simulink subsystem "controller_change"  (R2022b)
settings: Solver=VariableStepAuto  StartTime=0.0  StopTime=10.0  RelTol=1e-3
settings Model: Creator=Edp  LastModifiedBy=Edp

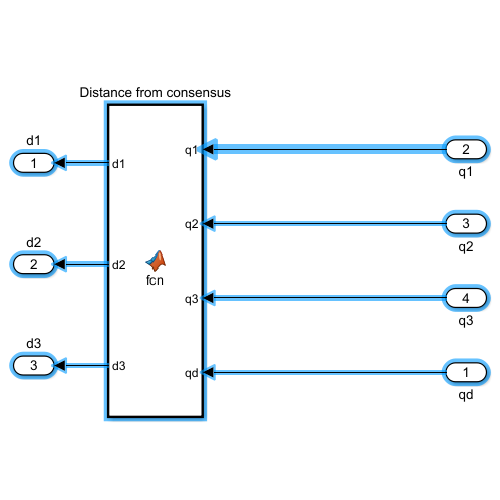
[thumbnail: Simulink's stored preview of the top-level diagram]
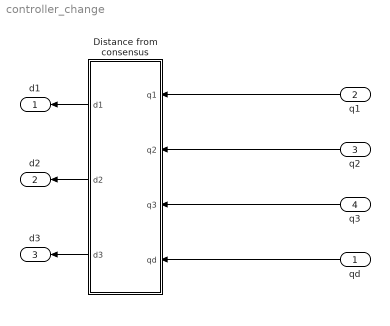
== system controller_change ==
  qd : Inport
  q1 : Inport  Port=2
  q2 : Inport  Port=3
  q3 : Inport  Port=4
  Distance from consensus : MATLAB Function  TreatAsAtomicUnit=on
  d1 : Outport
  d2 : Outport  Port=2
  d3 : Outport  Port=3
  wires:
  q2/1 -> Distance from consensus/2(q2)
  qd/1 -> Distance from consensus/4(qd)
  Distance from consensus/3(d3) -> d3/1
  q3/1 -> Distance from consensus/3(q3)
  Distance from consensus/1(d1) -> d1/1
  Distance from consensus/2(d2) -> d2/1
  q1/1 -> Distance from consensus/1(q1)

== matlab function controller_change/Distance from consensus ==
  data: q1 input; d1 output; q2 input; q3 input; qd input; d2 output; d3 output
function [d1, d2, d3] = fcn(q1,q2,q3,qd)

threshold = 4;

qq1 = [q1(1), q1(2)];
qq2 = [q2(1), q2(2)];
qq3 = [q3(1), q3(2)];
qqd = [qd(1), qd(2)];

err1 = norm(qq1 - qqd);
err2 = norm(qq2 - qqd);
err3 = norm(qq3 - qqd);

d1 = 1;
if err1 < threshold
    d1 = 0;
end

d2 = 1;
if err2 < threshold
    d2 = 0;
end

d3 = 1;
if err3 < threshold
    d3 = 0;
end
